simulink model "skijump_motor_test"  (R2024b)
settings: Solver=VariableStepAuto  StartTime=0.0  StopTime=1  RelTol=1e-3
model workspace (MAT data in the model file):
  Jb = 0.004
  Jr = 0.00105
  Kb = 0.2162
  Kt = 0.1573
  Ra = 2.264
  b = 0.01
  i_nl = 0.2
  omega_0 = 0
  v_ref = 12
libraries: simulink_extras x2
settings Model: Creator=f002r5k  LastModifiedBy=f002r5k

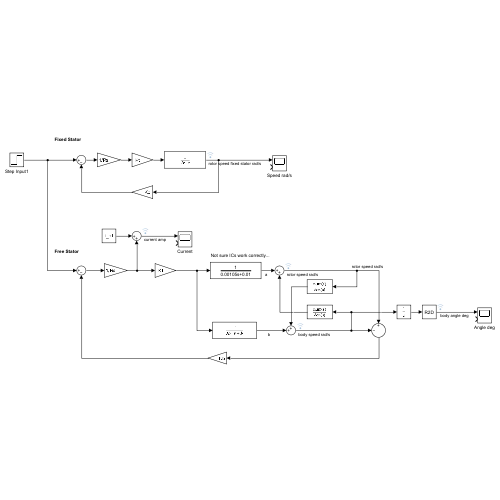
[thumbnail: Simulink's stored preview of the top-level diagram]
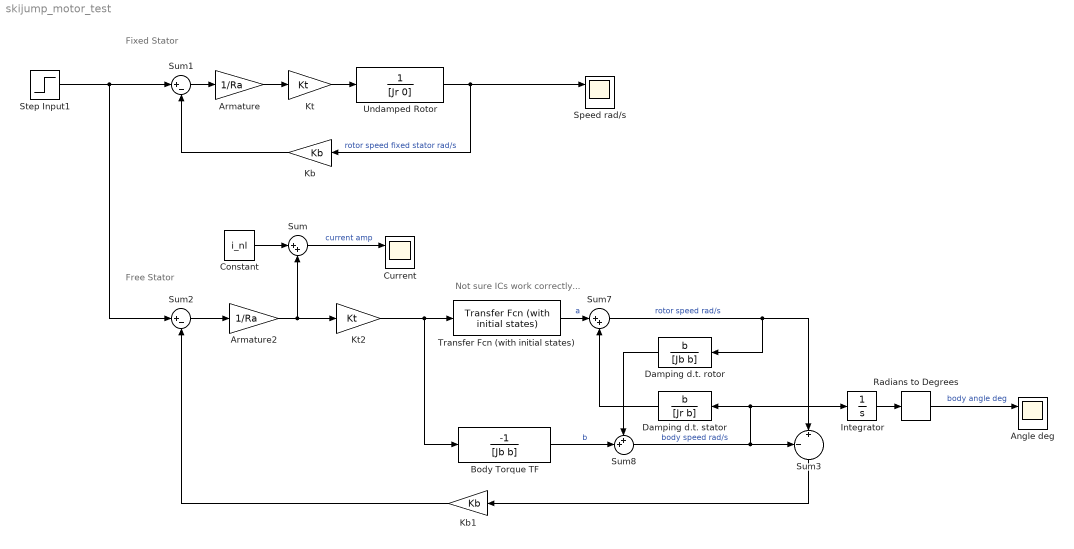
== system skijump_motor_test ==
  note: Fixed Stator
  note: Not sure ICs work correctly...
  note: Free Stator
  Angle deg : Scope  NumInputPorts=2
  Armature : Gain  Gain=1/Ra
  Armature2 : Gain  Gain=1/Ra
  Body Torque TF : TransferFcn  Numerator=-1  Denominator=[Jb b]
  Constant : Constant  Value=i_nl
  Current : Scope  NumInputPorts=2
  Damping d.t. rotor : TransferFcn  Numerator=b  Denominator=[Jb b]
  Damping d.t. stator : TransferFcn  Numerator=b  Denominator=[Jr b]
  Integrator : Integrator
  Kb : Gain  Gain=Kb
  Kb1 : Gain  Gain=Kb
  Kt : Gain  Gain=Kt
  Kt2 : Gain  Gain=Kt
  Radians to Degrees : simulink_extras/Transformations/Radians to Degrees
  Speed rad/s : Scope  NumInputPorts=2
  Step Input1 : Step  Time=0  Before=2  After=v_ref  SampleTime=0
  Sum : Sum  Inputs=|++
  Sum1 : Sum  Inputs=|+-
  Sum2 : Sum  Inputs=|+-
  Sum3 : Sum  Inputs=-|+||
  Sum7 : Sum  Inputs=|++
  Sum8 : Sum  Inputs=++|
  Transfer Fcn (with initial states) : simulink_extras/Additional Linear/Transfer Fcn (with initial states)  N=[1]  D=[Jr b]  X0=omega_0*Jr
  Undamped Rotor : TransferFcn  Numerator=1  Denominator=[Jr 0]
  wires:
  Sum1/1 -> Armature/1
  Armature/1 -> Kt/1
  Kt/1 -> Undamped Rotor/1
  Undamped Rotor/1 -> Speed rad/s/1, Kb/1  "rotor speed fixed stator rad/s"
  Kb/1 -> Sum1/2
  Kt2/1 -> Transfer Fcn (with initial states)/1, Body Torque TF/1
  Sum2/1 -> Armature2/1
  Armature2/1 -> Kt2/1, Sum/2
  Step Input1/1 -> Sum1/1, Sum2/1
  Constant/1 -> Sum/1
  Sum/1 -> Current/1  "current amp"
  Integrator/1 -> Radians to Degrees/1
  Radians to Degrees/1 -> Angle deg/1  "body angle deg"
  Transfer Fcn (with initial states)/1 -> Sum7/1  "a"
  Body Torque TF/1 -> Sum8/2  "b"
  Sum8/1 -> Sum3/1, Integrator/1, Damping d.t. stator/1  "body speed rad/s"
  Damping d.t. stator/1 -> Sum7/2
  Damping d.t. rotor/1 -> Sum8/1
  Sum3/1 -> Kb1/1
  Sum7/1 -> Sum3/2, Damping d.t. rotor/1  "rotor speed rad/s"
  Kb1/1 -> Sum2/2
